simulink model "ifelse"  (R2024a)
settings: Solver=VariableStepAuto  StartTime=0.0  StopTime=10.0  RelTol=1e-3
settings Model: Creator=Shuvo  LastModifiedBy=Shuvo

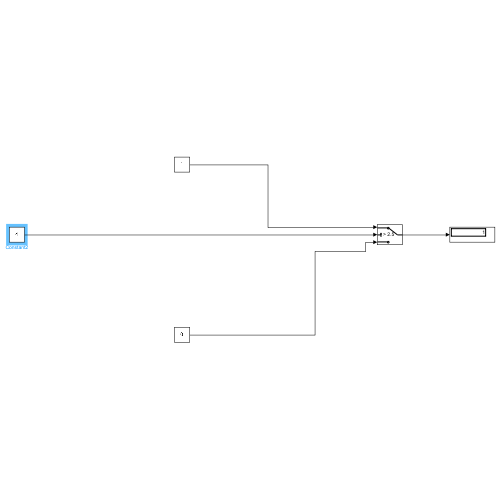
[thumbnail: Simulink's stored preview of the top-level diagram]
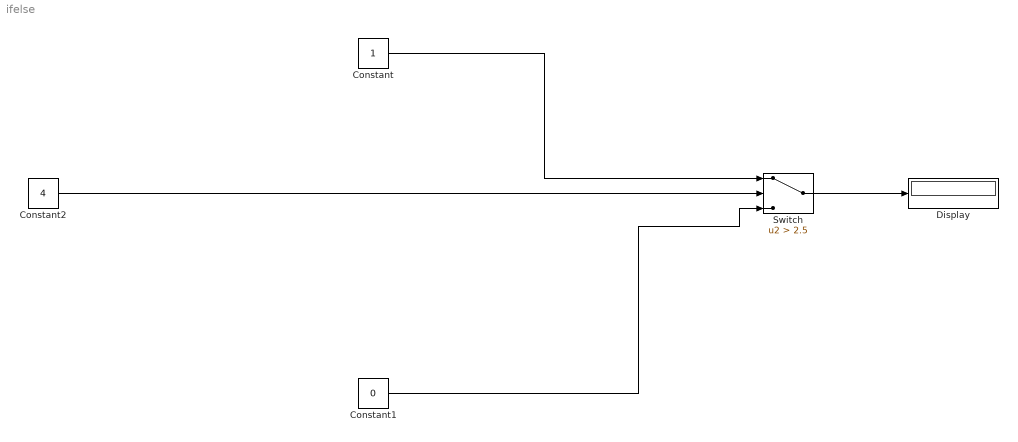
== system ifelse ==
  Constant : Constant
  Constant1 : Constant  Value=0
  Constant2 : Constant  Value=4
  Display : Display
  Switch : Switch  Criteria=u2 > Threshold  Threshold=2.5  SaturateOnIntegerOverflow=off  InputSameDT=off
  wires:
  Switch/1 -> Display/1
  Constant2/1 -> Switch/2
  Constant/1 -> Switch/1
  Constant1/1 -> Switch/3
